simulink model "heizung_example"  (R2020b)
settings: Solver=VariableStepAuto  StartTime=0.0  StopTime=60  RelTol=1e-3
InitFcn:
  | config
values from neighbouring files (symbols this model uses):
  A = 24    [config.m]
  alpha = 0.1    [config.m]
  C = 10    [config.m]
libraries: pid_lib x1
settings Model: EnablePacing=on  Creator=mateu  LastModifiedBy=mateu

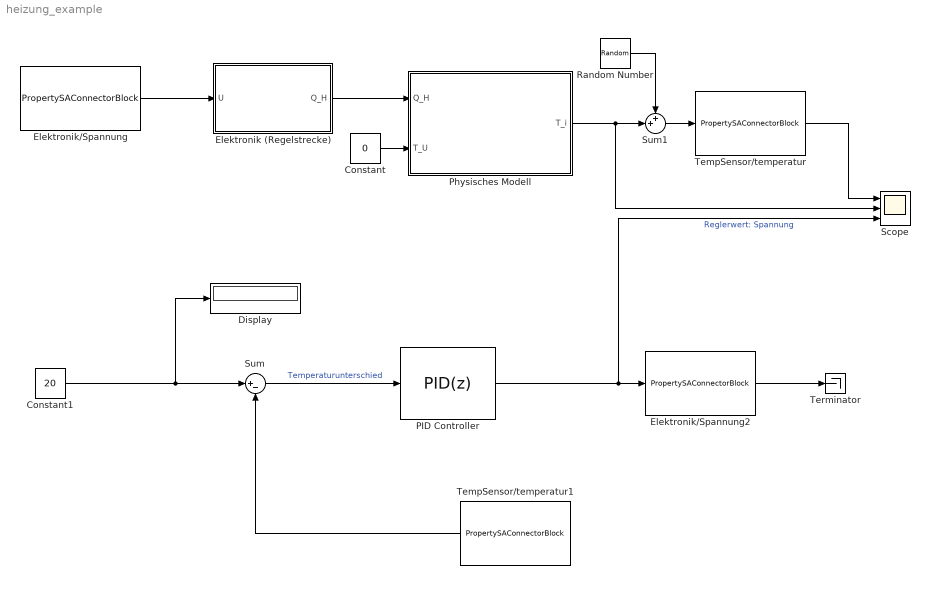
== system heizung_example ==
  Constant : Constant  Value=0
  Constant1 : Constant  Value=20
  Display : Display
  Elektronik (Regelstrecke) : Subsystem
  Elektronik/Spannung : S-Function  FunctionName=PropertySAConnectorBlock  Parameters=sr, regUrlStr, aasId, smId, seId  SFunctionDeploymentMode=off  EnableBusSupport=off  mask{sr=0.1, regUrlStr=http://localhost:8082/registry/api/v1/registrys, aasId=Test/Heizung/01, smId=Elektronik, seId=spannung}
      mask prompts: sr "Sample Rate"; regUrlStr "Registry URL"; aasId "AAS Id"; smId "Submodel IdShort"; seId "Property IdShort"
      mask DialogControl DescGroupVar Prompt: Standalone Property Block
      mask DialogControl DescTextVar Prompt: This block connects to a SubmodelElement running in an AAS Server. Data sent to the block's input updates the value of the SubmodelElement, whereas its current value is sent to the block's output. This process is repeated every sample rate interval.
      mask DialogControl Container4 Prompt: AAS Pars.
      mask DialogControl panelSE Prompt: SubmodelElement Pars.
      mask Display:
      | sr = get_param(gcb,'sr');
      | aas = get_param(gcb,'aasId');
      | sm = get_param(gcb,'smId');
      | se = get_param(gcb,'seId');
      | full = sm  + "/" + se;
      | 
      | pos = get_param(gcb, 'Position');
      | w = pos(3) - pos(1);
      | h = pos(4) - pos(2);
      | 
      | text(5,20, "{\bf\fontsize{7}"+aas+"}", 'texmode','on')
      | text(5,10, "{\bf\fontsize{6}"+full+"}", 'texmode','on')
      | image('basyx.png', [w-15,h-20,10,15]);
      | port_label('output', 1,"{\bf\fontsize{6}sr="+sr+"s}", 'texmode','on')
  Elektronik/Spannung2 : S-Function  FunctionName=PropertySAConnectorBlock  Parameters=sr, regUrlStr, aasId, smId, seId  SFunctionDeploymentMode=off  EnableBusSupport=off  mask{sr=0.25, regUrlStr=http://localhost:8082/registry/api/v1/registry, aasId=Test/Heizung/01, smId=Elektronik, seId=spannung}
      mask prompts: sr "Sample Rate"; regUrlStr "Registry URL"; aasId "AAS Id"; smId "Submodel IdShort"; seId "Property IdShort"
      mask Display:
      | sr = get_param(gcb,'sr')
      | aas = get_param(gcb,'aasId')
      | sm = get_param(gcb,'smId')
      | se = get_param(gcb,'seId')
      | 
      | pos = get_param(gcb, 'Position');
      | w = pos(3) - pos(1);
      | h = pos(4) - pos(2);
      | 
      | full = sm  + "/" + se
      | text(5,20, "{\bf\fontsize{7}"+aas+"}", 'texmode','on')
      | text(5,10, "{\bf\fontsize{6}"+full+"}", 'texmode','on')
      | image('basyx.png', [w-15,h-20,10,15]);
      | port_label('output', 1,"{\bf\fontsize{6}sr="+sr+"s}", 'texmode','on')
  PID Controller : pid_lib/PID Controller  Controller=PID  Form=Parallel  TimeDomain=Discrete-time  UseExternalTs=off  SampleTime=0.25  IntegratorMethod=Forward Euler  FilterMethod=Forward Euler  ControllerParametersSource=internal  P=0.3  I=0.1  D=0  UseFilter=off  N=100  TunerSelectOption=Transfer Function Based (PID Tuner App)  InitialConditionSource=internal  InitialConditionForIntegrator=0  InitialConditionForFilter=0  DifferentiatorICPrevScaledInput=0  ExternalReset=none  TrackingMode=off  Kt=1  LimitOutput=on  SatLimitsSource=internal  UpperSaturationLimit=10  LowerSaturationLimit=0  LinearizeAsGain=on  AntiWindupMode=none  Kb=1  POutMin=[]  POutMax=[]  IOutMin=[]  IOutMax=[]  DOutMin=[]  DOutMax=[]  NOutMin=[]  NOutMax=[]  SumOutMin=[]  SumOutMax=[]  SaturationOutMin=[]  SaturationOutMax=[]  PParamMin=[]  PParamMax=[]  IParamMin=[]  IParamMax=[]  DParamMin=[]  DParamMax=[]  NParamMin=[]  NParamMax=[]  KbParamMin=[]  KbParamMax=[]  KtParamMin=[]  KtParamMax=[]  KbOutMin=[]  KbOutMax=[]  KtOutMin=[]  KtOutMax=[]  IntegratorOutMin=[]  IntegratorOutMax=[]  FilterOutMin=[]  FilterOutMax=[]  SumI1OutMin=[]  SumI1OutMax=[]  SumI2OutMin=[]  SumI2OutMax=[]  SumI3OutMin=[]  SumI3OutMax=[]  SumI4OutMin=[]  SumI4OutMax=[]  SumDOutMin=[]  SumDOutMax=[]  DifferentiatorOutMin=[]  DifferentiatorOutMax=[]  FilterDiffOutCoefMin=[]  FilterDiffOutCoefMax=[]  ReciprocalOutMin=[]  ReciprocalOutMax=[]  SumDenOutMin=[]  SumDenOutMax=[]  SumNumOutMin=[]  SumNumOutMax=[]  DivideOutMin=[]  DivideOutMax=[]  UdiffTsProdOutMin=[]  UdiffTsProdOutMax=[]  NTsProdOutMin=[]  NTsProdOutMax=[]  UintegralTsProdOutMin=[]  UintegralTsProdOutMax=[]  UngainTsProdOutMin=[]  UngainTsProdOutMax=[]  IntegratorContinuousStateAttributes=''  IntegratorStateMustResolveToSignalObject=off  IntegratorRTWStateStorageClass=Auto  FilterContinuousStateAttributes=''  FilterStateMustResolveToSignalObject=off  FilterRTWStateStorageClass=Auto  ParallelPVariant=InternalParameters  IdealPVariant=Disabled  IVariant=InternalParameters  DVariant=InternalParameters  IntegratorVariant=Discrete  SatVariant=Enabled  AWVariant=Passthrough  PCopyVariant=Disabled  TRVariant=Disabled  FdbkBlocksVariant=Forward  IdealPFdbkVariant=Disabled  SatFdbkVariant=Disabled  DerivativeFilterVariant=Differentiator  NVariant=Passthrough  NCopyVariant=Disabled_SignalSpec  FilterICVariant=InternalICsDifferentiator  IntegratorICVariant=InternalICs  ExternalResetVariant=Disabled  TRSumVariant=Passthrough  SumFdbkVariant=Disabled  SumVariant=Sum_PID  TsampFilterVariant=InternalTs  TsampNgainVariant=Passthrough  TsampIntegralVariant=Passthrough  ExternalSaturationOutDataTypeStr=Inherit: Same as second input
  Physisches Modell : Subsystem
  Random Number : RandomNumber  Variance=0.25  Seed=12313  SampleTime=0.1
  Scope : Scope  NumInputPorts=3
  Sum : Sum  Inputs=|+-
  Sum1 : Sum  Inputs=++|
  TempSensor/temperatur : S-Function  FunctionName=PropertySAConnectorBlock  Parameters=sr, regUrlStr, aasId, smId, seId  SFunctionDeploymentMode=off  EnableBusSupport=off  mask{sr=1, regUrlStr=http://localhost:8082/registry/api/v1/registry, aasId=Test/Heizung/01, smId=TempSensor, seId=temperatur}
      mask prompts: sr "Sample Rate"; regUrlStr "Registry URL"; aasId "AAS Id"; smId "Submodel IdShort"; seId "Property IdShort"
      mask Display:
      | sr = get_param(gcb,'sr')
      | aas = get_param(gcb,'aasId')
      | sm = get_param(gcb,'smId')
      | se = get_param(gcb,'seId')
      | 
      | pos = get_param(gcb, 'Position');
      | w = pos(3) - pos(1);
      | h = pos(4) - pos(2);
      | 
      | full = sm  + "/" + se
      | text(5,20, "{\bf\fontsize{7}"+aas+"}", 'texmode','on')
      | text(5,10, "{\bf\fontsize{6}"+full+"}", 'texmode','on')
      | image('basyx.png', [w-15,h-20,10,15]);
      | port_label('output', 1,"{\bf\fontsize{6}sr="+sr+"s}", 'texmode','on')
  TempSensor/temperatur1 : S-Function  FunctionName=PropertySAConnectorBlock  Parameters=sr, regUrlStr, aasId, smId, seId  SFunctionDeploymentMode=off  EnableBusSupport=off  mask{sr=1, regUrlStr=http://localhost:8082/registry/api/v1/registry, aasId=Test/Heizung/01, smId=TempSensor, seId=temperatur}
      mask prompts: sr "Sample Rate"; regUrlStr "Registry URL"; aasId "AAS Id"; smId "Submodel IdShort"; seId "Property IdShort"
      mask Display:
      | sr = get_param(gcb,'sr')
      | aas = get_param(gcb,'aasId')
      | sm = get_param(gcb,'smId')
      | se = get_param(gcb,'seId')
      | 
      | pos = get_param(gcb, 'Position');
      | w = pos(3) - pos(1);
      | h = pos(4) - pos(2);
      | 
      | full = sm  + "/" + se
      | text(5,20, "{\bf\fontsize{7}"+aas+"}", 'texmode','on')
      | text(5,10, "{\bf\fontsize{6}"+full+"}", 'texmode','on')
      | image('basyx.png', [w-15,h-20,10,15]);
      | port_label('output', 1,"{\bf\fontsize{6}sr="+sr+"s}", 'texmode','on')
  Terminator : Terminator
  wires:
  Constant/1 -> Physisches Modell/2(T_U)
  Physisches Modell/1(T_i) -> Sum1/2, Scope/2
  TempSensor/temperatur/1 -> Scope/1
  Elektronik (Regelstrecke)/1(Q_H) -> Physisches Modell/1(Q_H)
  Elektronik/Spannung/1 -> Elektronik (Regelstrecke)/1(U)
  PID Controller/1 -> Elektronik/Spannung2/1, Scope/3  "Reglerwert: Spannung"
  Constant1/1 -> Display/1, Sum/1
  Sum/1 -> PID Controller/1  "Temperaturunterschied"
  TempSensor/temperatur1/1 -> Sum/2
  Random Number/1 -> Sum1/1
  Sum1/1 -> TempSensor/temperatur/1
  Elektronik/Spannung2/1 -> Terminator/1

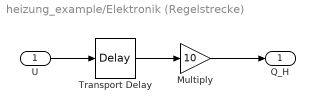
== system heizung_example/Elektronik (Regelstrecke) ==
  U : Inport
  Multiply : Gain  Gain=10
  Transport Delay : TransportDelay
  Q_H : Outport
  wires:
  Multiply/1 -> Q_H/1
  U/1 -> Transport Delay/1
  Transport Delay/1 -> Multiply/1

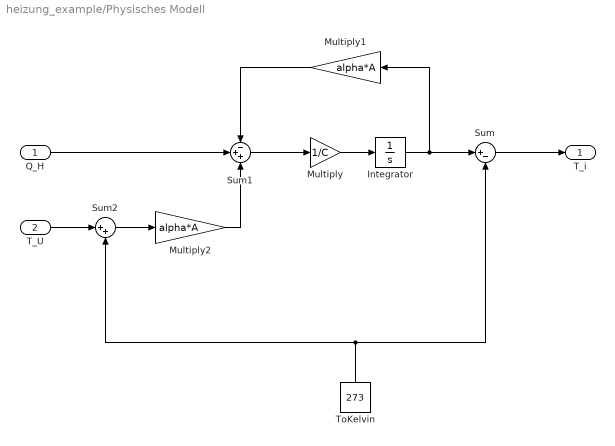
== system heizung_example/Physisches Modell ==
  Q_H : Inport
  T_U : Inport  Port=2
  Integrator : Integrator  InitialCondition=273
  Multiply : Gain  Gain=1/C
  Multiply1 : Gain  Gain=alpha*A
  Multiply2 : Gain  Gain=alpha*A
  Sum : Sum  Inputs=|+-
  Sum1 : Sum  Inputs=-++
  Sum2 : Sum  Inputs=|++
  ToKelvin : Constant  Value=273
  T_i : Outport
  wires:
  T_U/1 -> Sum2/1
  Integrator/1 -> Sum/1, Multiply1/1
  Q_H/1 -> Sum1/2
  Multiply1/1 -> Sum1/1
  ToKelvin/1 -> Sum/2, Sum2/2
  Multiply/1 -> Integrator/1
  Multiply2/1 -> Sum1/3
  Sum1/1 -> Multiply/1
  Sum2/1 -> Multiply2/1
  Sum/1 -> T_i/1
